simulink model "pressingswitch_fan_stateflow"  (R2021a)
settings: Solver=VariableStepAuto  StartTime=0.0  StopTime=inf  RelTol=1e-3
settings Model: Creator=surya  LastModifiedBy=surya

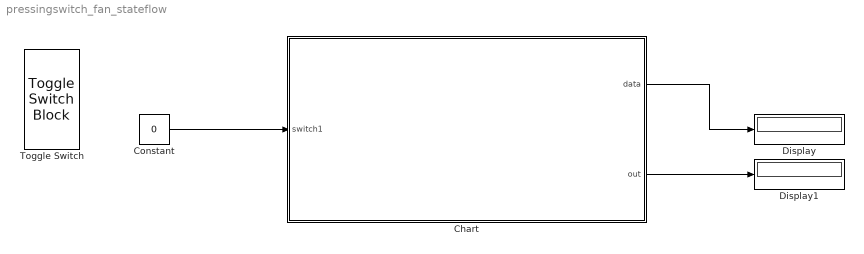
== system pressingswitch_fan_stateflow ==
  Chart : Stateflow chart  TreatAsAtomicUnit=on
  Constant : Constant  Value=0
  Display : Display
  Display1 : Display
  Toggle Switch : ToggleSwitchBlock
      settings: Values={{'Off', 'On'}, [0 1]}
  wires:
  Chart/1(data) -> Display/1
  Chart/2(out) -> Display1/1
  Constant/1 -> Chart/1(switch1)

== stateflow chart pressingswitch_fan_stateflow/Chart ==
  state counter2(y) [function]
    (default) -> (junction 2)
    (junction 2) -> (junction 1) : {t=y}
    (junction 1) -> (junction 3) [order 1] : [switch1==1& t<500]
    (junction 4) -> (junction 1)
    (junction 1) -> (junction 5) [order 2] : {data=t}
    (junction 3) -> (junction 4) : {t=t+1}
  state off
    en:
    out=0
  state on
    en:
    out=1
  (default) -> off
  off -> (junction 28) : [switch1==1]{counter2(0)}
  (junction 28) -> on : [switch1==1& data>=500]
  on -> off : [switch1==0]{data=0}
  data: y function_input; data output; t local; out output; switch1 input
